simulink model "DC_moteor_fdi1"  (R2024b)
settings: Solver=VariableStepAuto  StartTime=0.0  StopTime=inf  RelTol=1e-3
values from neighbouring files (symbols this model uses):
  Af = 0.01    [Data__MOTOR.m]    (also in Generator_Data.m = 0.0001; Generator_Datatest.m)
  Bf = 0.0002    [Data__MOTOR.m]    (also in Generator_Data.m = 2e-05; Generator_Datatest.m)
  Cc = Cc0+6*Cc0    (= 0.7)    [Data__MOTOR.m]    (also in Generator_Datatest.m)
  Cc0 = 0.1    [Data__MOTOR.m]    (also in Generator_Datatest.m)
  CurrentFaultSwitch = 0    [Data__MOTOR.m]    (also in Generator_Data.m = 1; Generator_Datatest.m)
  Jm = 0.08    [Data__MOTOR.m]    (also in Generator_Datatest.m)
  Ke = 0.139    [Data__MOTOR.m]    (also in Generator_Datatest.m)
  Le = 0.44    [Data__MOTOR.m]    (also in Generator_Datatest.m)
  rate_noise_i = 0.02*In    (= 0.22)    [Data__MOTOR.m]    (also in Generator_Data.m = 0.02; Generator_Datatest.m)
  rate_noise_w = 0.02*Wn    (= 2.96)    [Data__MOTOR.m]    (also in Generator_Data.m = 0.002; Generator_Datatest.m)
  Re = 2.4    [Data__MOTOR.m]    (also in Generator_Datatest.m)
  ResFaultSwitch = 0    [Data__MOTOR.m]    (also in Generator_Datatest.m)
  Rm = 0.01    [Data__MOTOR.m]    (also in Generator_Datatest.m)
  StartStop = 0    [Data__MOTOR.m]    (also in Generator_Data.m; Generator_Datatest.m)
  Te = 0.1    [Data__MOTOR.m]    (also in Generator_Data.m = 1; Generator_Datatest.m)
  Ua = 48    [Data__MOTOR.m]    (also in Generator_Datatest.m)
  VelocityFaultSwitch = 0    [Data__MOTOR.m]    (also in Generator_Data.m = 1; Generator_Datatest.m)
undefined symbols (not defined in the file or in its folder): dspblkCoreblockFVToolHelper, gcbh, sigbuilder_block
libraries: SignalEditorBlockLib x2
(part 3 of 3)

== system DC_moteor_fdi1/HOME ==

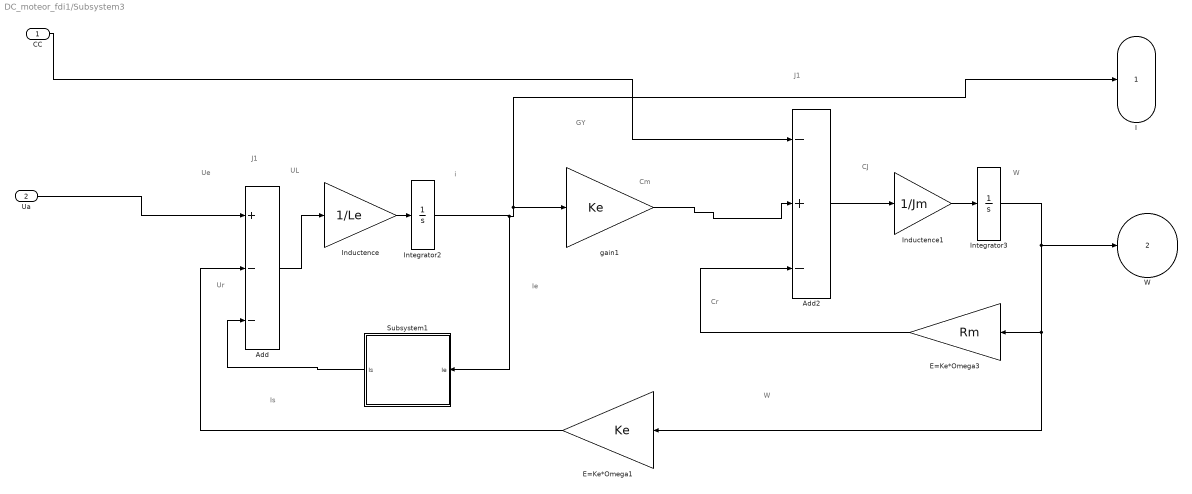
== system DC_moteor_fdi1/Subsystem3 ==
  note: J1
  note: i
  note: GY
  note: J1
  note: UL
  note: Ue
  note: Cr
  note: W
  note: Cm
  note: CJ
  note: Ur
  note: W
  note: Is
  note: Ie
  CC : Inport
  Ua : Inport  Port=2
  Add : Sum  Inputs=+--
  Add2 : Sum  Inputs=-+-
  E=Ke*Omega1 : Gain  Gain=Ke
  E=Ke*Omega3 : Gain  Gain=Rm
  Inductence : Gain  Gain=1/Le
  Inductence1 : Gain  Gain=1/Jm
  Integrator2 : Integrator
  Integrator3 : Integrator
  Subsystem1 : Subsystem
      mask Display: disp('Re')
  gain1 : Gain  Gain=Ke
  I : Outport
  W : Outport  Port=2
  wires:
  E=Ke*Omega3/1 -> Add2/3
  gain1/1 -> Add2/2
  Integrator3/1 -> E=Ke*Omega3/1, E=Ke*Omega1/1, W/1
  Ua/1 -> Add/1
  Integrator2/1 -> Subsystem1/1(Ie), I/1, gain1/1
  Subsystem1/1(Is) -> Add/3
  Inductence/1 -> Integrator2/1
  Add2/1 -> Inductence1/1
  Add/1 -> Inductence/1
  Inductence1/1 -> Integrator3/1
  E=Ke*Omega1/1 -> Add/2
  CC/1 -> Add2/1

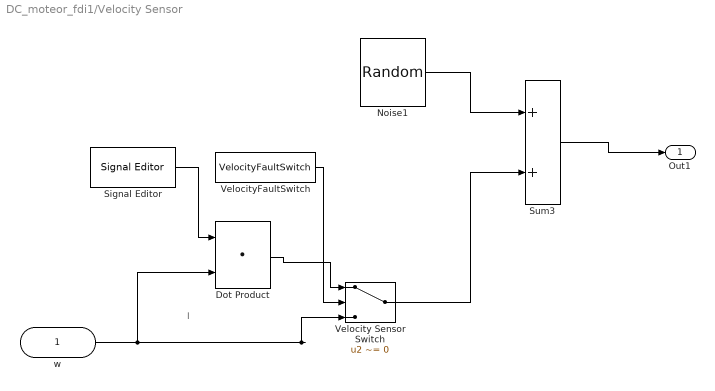
== system DC_moteor_fdi1/Velocity Sensor ==
  note: I
  w : Inport
  Dot Product : DotProduct  OutDataTypeStr=Inherit: Inherit via internal rule
  Noise1 : UniformRandomNumber  Minimum=-rate_noise_w  Maximum=+rate_noise_w  SampleTime=0.1
  Signal Editor : SignalEditorBlockLib/Signal Editor  FileName=VelocityFault.mat  ActiveScenario=ChuteVelocite  ActiveSignal=Fault  IsBus=off  OutputBusObjectStr=Bus: BusObject  SampleTime=0  Interpolate=off  ZeroCross=off  OutputAfterFinalValue=Setting to zero  Unit=inherit  PreserveSignalName=on  ApplySigPropsToAllScenarios=on  ApplySigPropsToAllSignals=off
  Sum3 : Sum  InputSameDT=on  SaturateOnIntegerOverflow=on  OutDataTypeStr=Inherit: Same as first input
  Velocity Sensor Switch : Switch  Criteria=u2 ~= 0  Threshold=1  SaturateOnIntegerOverflow=off  InputSameDT=off
  VelocityFaultSwitch : Constant  Value=VelocityFaultSwitch
  Out1 : Outport  VectorParamsAs1DForOutWhenUnconnected=off
  wires:
  Sum3/1 -> Out1/1
  w/1 -> Dot Product/2, Velocity Sensor Switch/3
  Signal Editor/1 -> Dot Product/1
  Dot Product/1 -> Velocity Sensor Switch/1
  Velocity Sensor Switch/1 -> Sum3/2
  Noise1/1 -> Sum3/1
  VelocityFaultSwitch/1 -> Velocity Sensor Switch/2

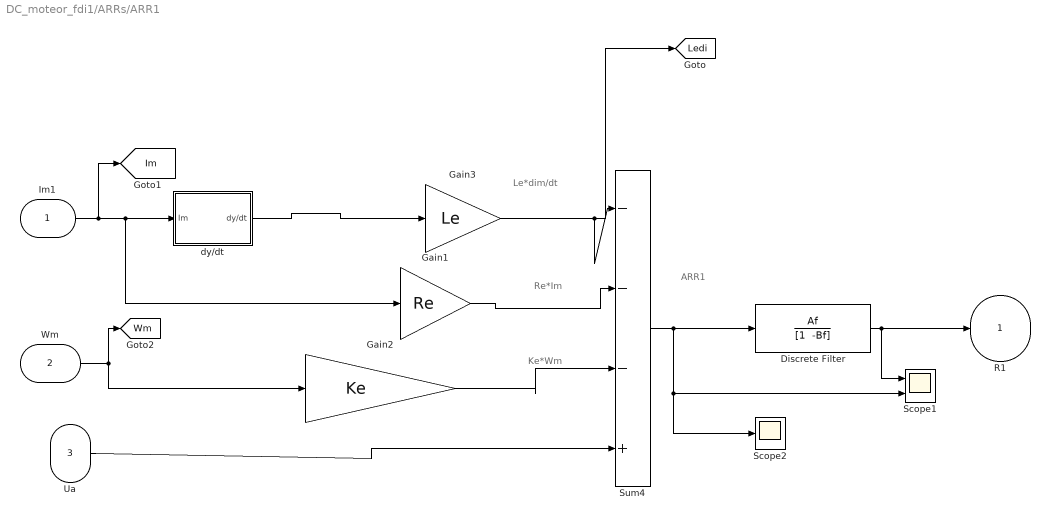
== system DC_moteor_fdi1/ARRs/ARR1 ==
  note: ARR1
  note: Re*Im
  note: Le*dim/dt
  note: Ke*Wm
  Im1 : Inport
  Wm : Inport  Port=2
  " Ua" : Inport  Port=3
  Discrete Filter : DiscreteFilter  LoadFcn=dspblkCoreblockFVToolHelper(gcbh,'load');  Numerator=Af  Denominator="[1  -Bf]"  SampleTime=Te  a0EqualsOne=on
      settings: CopyFcn=dspblkCoreblockFVToolHelper(gcbh,'copy');  DeleteFcn=dspblkCoreblockFVToolHelper(gcbh,'close');  ModelCloseFcn=dspblkCoreblockFVToolHelper(gcbh,'close');  PreSaveFcn=dspblkCoreblockFVToolHelper(gcbh,'presave');  PostSaveFcn=dspblkCoreblockFVToolHelper(gcbh,'postsave');  CloseFcn=dspblkCoreblockFVToolHelper(gcbh,'close');
  Gain1 : Gain  Gain=Re
  Gain2 : Gain  Gain=Ke
  Gain3 : Gain  Gain=Le
  Scope1 : Scope  NumInputPorts=2
  Scope2 : Scope
  Sum4 : Sum  Inputs=|---+
  dy/dt : Subsystem
  R1 : Outport  VectorParamsAs1DForOutWhenUnconnected=off
  tag scope: Im=global, Ledi=global, Wm=global
  wires:
  Gain1/1 -> Sum4/2
  Wm/1 -> [Wm], Gain2/1
  Gain2/1 -> Sum4/3
  " Ua"/1 -> Sum4/4
  Im1/1 -> [Im], dy/dt/1(Im), Gain1/1
  Gain3/1 -> [Ledi], Sum4/1
  dy/dt/1(dy/dt) -> Gain3/1
  Sum4/1 -> Discrete Filter/1, Scope1/2, Scope2/1
  Discrete Filter/1 -> R1/1, Scope1/1

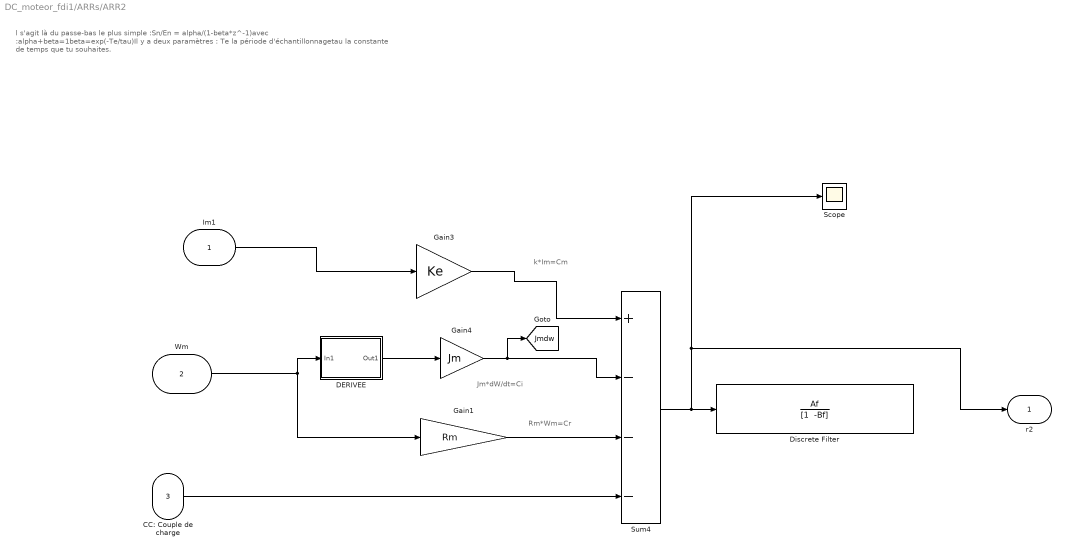
== system DC_moteor_fdi1/ARRs/ARR2 ==
  note: l s'agit là du passe-bas le plus simple :Sn/En = alpha/(1-beta*z^-1)avec :alpha+beta=1beta=exp(-Te/tau)Il y a deux paramètres : Te la période d'échantillonnagetau la constante de temps que tu souhaites.
  note: Rm*Wm=Cr
  note: k*Im=Cm
  note: Jm*dW/dt=Ci
  Im1 : Inport
  Wm : Inport  Port=2
  CC: Couple de charge : Inport  Port=3
  DERIVEE : Subsystem
  Discrete Filter : DiscreteFilter  LoadFcn=dspblkCoreblockFVToolHelper(gcbh,'load');  Numerator=Af  Denominator="[1  -Bf]"  SampleTime=Te  a0EqualsOne=on
      settings: CopyFcn=dspblkCoreblockFVToolHelper(gcbh,'copy');  DeleteFcn=dspblkCoreblockFVToolHelper(gcbh,'close');  ModelCloseFcn=dspblkCoreblockFVToolHelper(gcbh,'close');  PreSaveFcn=dspblkCoreblockFVToolHelper(gcbh,'presave');  PostSaveFcn=dspblkCoreblockFVToolHelper(gcbh,'postsave');  CloseFcn=dspblkCoreblockFVToolHelper(gcbh,'close');
  Gain1 : Gain  Gain=Rm
  Gain3 : Gain  Gain=Ke
  Gain4 : Gain  Gain=Jm
  Scope : Scope
  Sum4 : Sum  Inputs=+---
  r2 : Outport  VectorParamsAs1DForOutWhenUnconnected=off
  tag scope: Jmdw=global
  wires:
  Im1/1 -> Gain3/1
  Gain4/1 -> [Jmdw], Sum4/2
  CC: Couple de charge/1 -> Sum4/4
  Gain1/1 -> Sum4/3
  Wm/1 -> Gain1/1, DERIVEE/1(In1)
  Sum4/1 -> r2/1, Scope/1, Discrete Filter/1
  DERIVEE/1(Out1) -> Gain4/1
  Gain3/1 -> Sum4/1

== system DC_moteor_fdi1/Dashboard/Initialisation ==

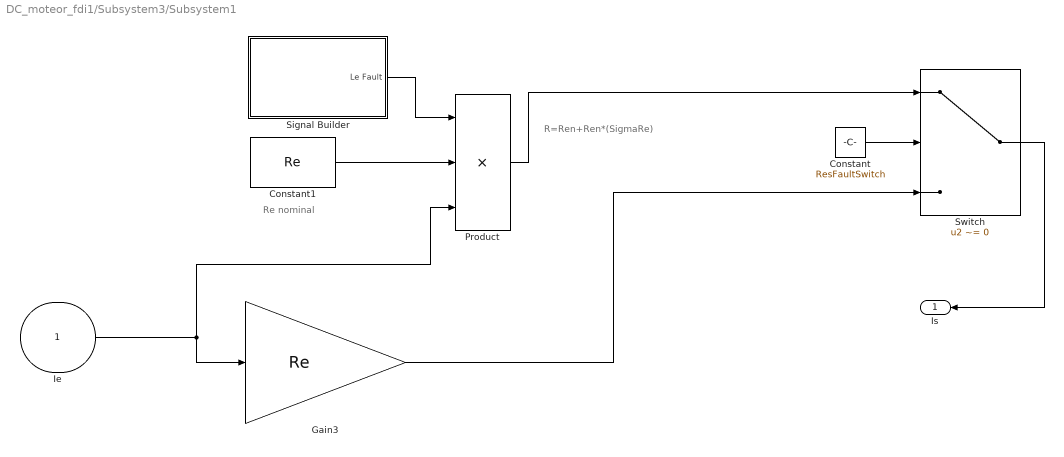
== system DC_moteor_fdi1/Subsystem3/Subsystem1 ==
  note: Re nominal
  note: R=Ren+Ren*(SigmaRe)
  Ie : Inport
  Constant : Constant  Value=ResFaultSwitch
  Constant1 : Constant  Value=Re
  Gain3 : Gain  Gain=Re
  Product : Product  Inputs=3
  Signal Builder : Subsystem  Tag=STV Subsys  LoadFcn=sigbuilder_block('load');  StartFcn=sigbuilder_block('start');  StopFcn=sigbuilder_block('stop');  ClipboardFcn=sigbuilder_block('clipboard');  mask(Sigbuilder block){tuvar=[0:10]}
      mask help: Simulink:masks:SigbuilderBlock_MD
      mask init:
      | if ~strcmp(get_param(bdroot(gcbh),'SimulationStatus'),'stopped') tuvar = sigbuilder_block('maskInit'); end
      settings: CopyFcn=sigbuilder_block('copy');  DeleteFcn=sigbuilder_block('delete');  ModelCloseFcn=sigbuilder_block('modelClose');  PreSaveFcn=sigbuilder_block('preSave');  PauseFcn=sigbuilder_block('pause');  ContinueFcn=sigbuilder_block('continue');  NameChangeFcn=sigbuilder_block('namechange');  OpenFcn=sigbuilder_block('open',[122.4 104 1024.2 446.8 ]);  CloseFcn=sigbuilder_block('close');
      mask Display: plot(0, 0, 100, 100,[2, 2, 32, 32, 2], [68, 8, 8, 68, 68],[32, 2], [38, 38], [32, 19, 2],[53, 60, 44], [32, 17, 17, 2],[16, 16, 31, 31]);txt = getActiveGroup(gcbh);text(2, 100, txt,'verticalAlignment', 'top');
  Switch : Switch  Criteria=u2 ~= 0  Threshold=1  SaturateOnIntegerOverflow=off  InputSameDT=off
  Is : Outport
  wires:
  Product/1 -> Switch/1
  Gain3/1 -> Switch/3
  Constant1/1 -> Product/2
  Signal Builder/1(Le Fault) -> Product/1
  Ie/1 -> Gain3/1, Product/3
  Constant/1 -> Switch/2
  Switch/1 -> Is/1

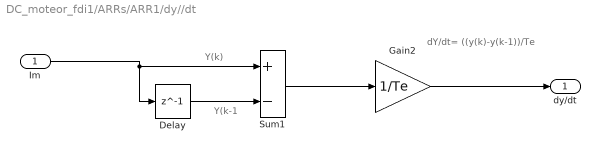
== system DC_moteor_fdi1/ARRs/ARR1/dy//dt ==
  note: dY/dt= ((y(k)-y(k-1))/Te
  note: Y(k)
  note: Y(k-1
  Im : Inport
  Delay : Delay  DelayLength=1  SampleTime=Te
  Gain2 : Gain  Gain=1/Te
  Sum1 : Sum  Inputs=+-
  dy/dt : Outport  VectorParamsAs1DForOutWhenUnconnected=off
  wires:
  Gain2/1 -> dy/dt/1
  Sum1/1 -> Gain2/1
  Delay/1 -> Sum1/2
  Im/1 -> Delay/1, Sum1/1

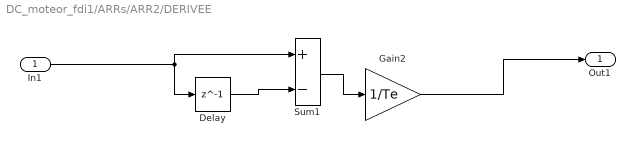
== system DC_moteor_fdi1/ARRs/ARR2/DERIVEE ==
  In1 : Inport
  Delay : Delay  DelayLength=1  SampleTime=Te
  Gain2 : Gain  Gain=1/Te
  Sum1 : Sum  Inputs=+-
  Out1 : Outport  VectorParamsAs1DForOutWhenUnconnected=off
  wires:
  In1/1 -> Sum1/1, Delay/1
  Delay/1 -> Sum1/2
  Sum1/1 -> Gain2/1
  Gain2/1 -> Out1/1

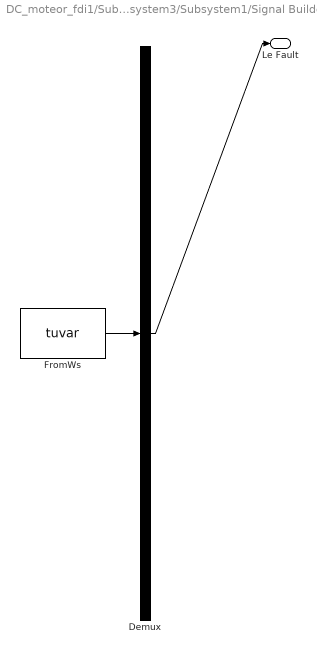
== system DC_moteor_fdi1/Subsystem3/Subsystem1/Signal Builder ==
  Demux : Demux  Tag=STV Demux  Outputs=1
      settings: DisplayOption=none
  FromWs : FromWorkspace  Tag=STV FromWs  VariableName=tuvar
      SigBuilderData=|
      | common.afterFinalStr = 'Extrapolate'
      | common.sampleTime = 0
      | dataSet.timeRange = [0 200]
      | dataSet.name = 'Group 1'
      | sbobj.Groups.Name = 'Group 1'
      | sbobj.Groups.Signals.Name = 'Le Fault'
      | sbobj.Groups.Signals.XData = [0 53.6 53.6 80.8 80.8 119.5 144 162.5 164.5 181.6 200]
      | sbobj.Groups.Signals.YData = [1 1 0.898 0.841 1 1 1 1 1 1 1]
      | sbobj.Groups.TimeRange = [0 200]
  Le Fault : Outport  Tag=STV Outport  VectorParamsAs1DForOutWhenUnconnected=off
  wires:
  FromWs/1 -> Demux/1
  Demux/1 -> Le Fault/1
